simulink model "guidance_2016"  (R2016b)
settings: Solver=VariableStepAuto  StartTime=0.0  StopTime=1000.0  RelTol=1e-3
libraries: marine_gnc x1
settings Model: Creator=mikkelsorensen  LastModifiedBy=mikkelsorensen

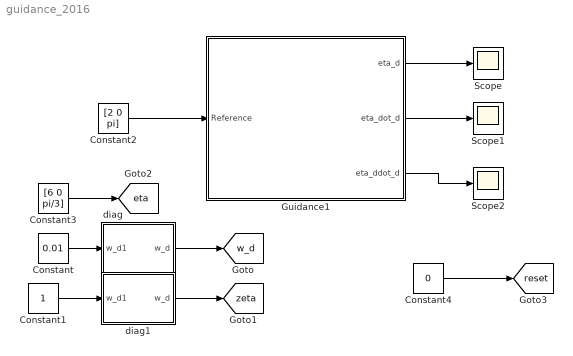
== system guidance_2016 ==
  Constant : Constant  Value=0.01
  Constant1 : Constant
  Constant2 : Constant  Value=[2 0 pi]
  Constant3 : Constant  Value=[6 0 pi/3]
  Constant4 : Constant  Value=0
  Guidance1 : Subsystem
  Scope : Scope
  Scope1 : Scope
  Scope2 : Scope
  diag : MATLAB Function  TreatAsAtomicUnit=on
  diag1 : MATLAB Function  TreatAsAtomicUnit=on
  tag scope: eta=global, reset=global, w_d=global, zeta=global
  wires:
  Constant/1 -> diag/1(w_d1)
  Constant1/1 -> diag1/1(w_d1)
  Constant2/1 -> Guidance1/1("Reference ")
  Constant3/1 -> [eta]
  Constant4/1 -> [reset]
  diag/1(w_d) -> [w_d]
  diag1/1(w_d) -> [zeta]
  Guidance1/1(eta_d) -> Scope/1
  Guidance1/3(eta_ddot_d) -> Scope2/1
  Guidance1/2(eta_dot_d) -> Scope1/1

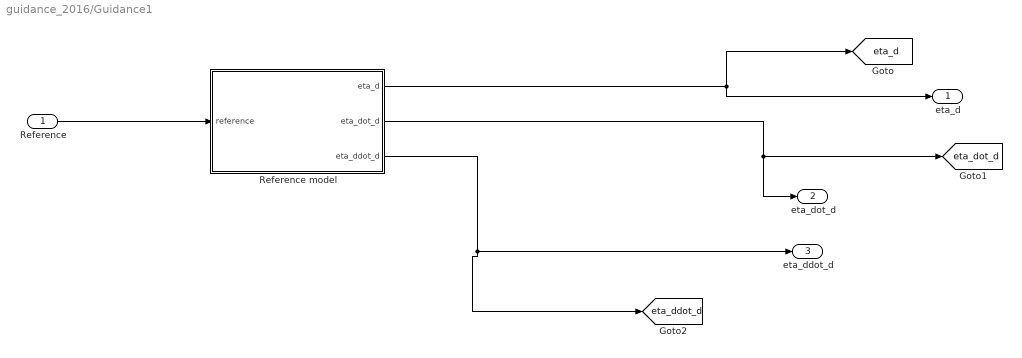
== system guidance_2016/Guidance1 ==
  "Reference " : Inport
  Reference model : Subsystem
  eta_d : Outport
  eta_dot_d : Outport  Port=2
  eta_ddot_d : Outport  Port=3
  tag scope: eta_d=global, eta_ddot_d=global, eta_dot_d=global
  wires:
  Reference model/1(eta_d) -> [eta_d], eta_d/1
  Reference model/2(eta_dot_d) -> eta_dot_d/1, [eta_dot_d]
  Reference model/3(eta_ddot_d) -> [eta_ddot_d], eta_ddot_d/1
  "Reference "/1 -> Reference model/1(reference)

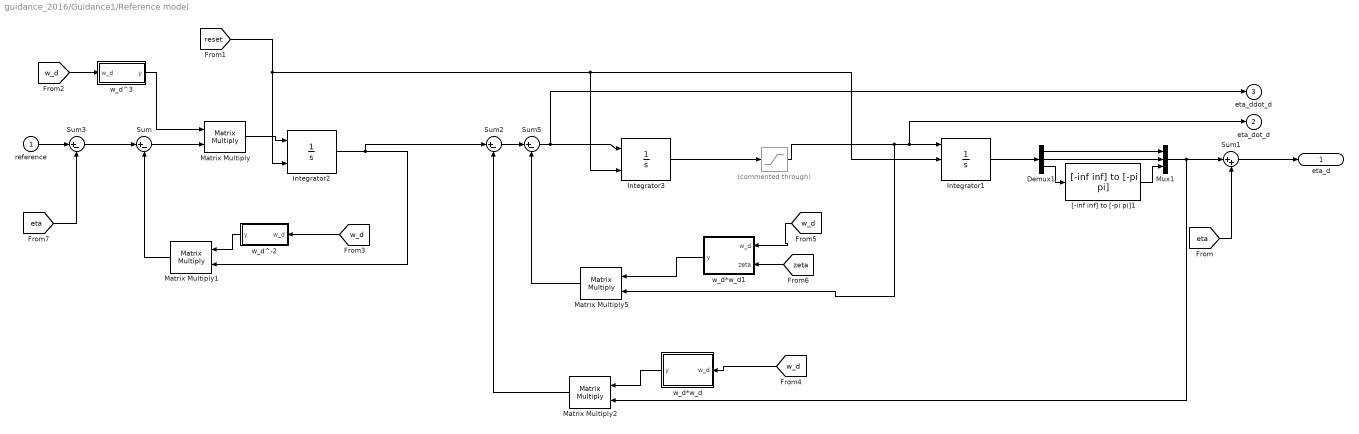
== system guidance_2016/Guidance1/Reference model ==
  reference : Inport
  "       " : Saturate  Commented=through  UpperLimit=[0.3 0.1 1]  LowerLimit=-[0.3 0.1 1]
  Demux1 : Demux  Outputs=3
  Integrator1 : Integrator  ExternalReset=either  InitialConditionSource=external
  Integrator2 : Integrator  ExternalReset=either
  Integrator3 : Integrator  ExternalReset=either
  Matrix Multiply{,1..2,5} (4 alike) : Product  Multiplication=Matrix(*)
  Mux1 : Mux  Inputs=3
  Sum : Sum  Inputs=|+-
  Sum1 : Sum  Inputs=|++  SaturateOnIntegerOverflow=on  InputSameDT=on  OutDataTypeStr=Inherit: Same as first input
  Sum2 : Sum  Inputs=|+-  SaturateOnIntegerOverflow=on  InputSameDT=on  OutDataTypeStr=Inherit: Same as first input
  Sum3 : Sum  Inputs=|+-  SaturateOnIntegerOverflow=on  InputSameDT=on  OutDataTypeStr=Inherit: Same as first input
  Sum5 : Sum  Inputs=|+-  SaturateOnIntegerOverflow=on  InputSameDT=on  OutDataTypeStr=Inherit: Same as first input
  "[-inf inf] to [-pi pi]1" : marine_gnc/Utilities/Math Operations/[-inf inf] to [-pi pi]
  w_d*w_d : MATLAB Function  TreatAsAtomicUnit=on
  w_d*w_d1 : MATLAB Function  TreatAsAtomicUnit=on
  w_d^-2 : MATLAB Function  TreatAsAtomicUnit=on
  w_d^3 : MATLAB Function  TreatAsAtomicUnit=on
  eta_d : Outport  InitialOutput=0
  eta_dot_d : Outport  Port=2  InitialOutput=0
  eta_ddot_d : Outport  Port=3  InitialOutput=0
  wires:
  "       "/1 -> eta_dot_d/1, Integrator1/1, Matrix Multiply5/2
  Sum5/1 -> Integrator3/1, eta_ddot_d/1
  Integrator2/1 -> Sum2/1, Matrix Multiply1/2
  Sum2/1 -> Sum5/1
  Matrix Multiply2/1 -> Sum2/2
  Mux1/1 -> Sum1/1, Matrix Multiply2/2
  Integrator3/1 -> "       "/1
  Matrix Multiply5/1 -> Sum5/2
  Sum/1 -> Matrix Multiply/2
  Matrix Multiply/1 -> Integrator2/1
  Matrix Multiply1/1 -> Sum/2
  [w_d] -> w_d^3/1(w_d)
  [w_d] -> w_d^-2/1(w_d)
  [w_d] -> w_d*w_d/1(w_d)
  w_d*w_d/1(y) -> Matrix Multiply2/1
  [zeta] -> w_d*w_d1/2(zeta)
  [w_d] -> w_d*w_d1/1(w_d)
  w_d*w_d1/1(y) -> Matrix Multiply5/1
  [reset] -> Integrator3/2, Integrator1/2, Integrator2/2
  w_d^-2/1(y) -> Matrix Multiply1/1
  w_d^3/1(y) -> Matrix Multiply/1
  Demux1/1 -> Mux1/1
  "[-inf inf] to [-pi pi]1"/1 -> Mux1/3
  Demux1/3 -> "[-inf inf] to [-pi pi]1"/1
  Demux1/2 -> Mux1/2
  Integrator1/1 -> Demux1/1
  [eta] -> Sum1/2
  Sum1/1 -> eta_d/1
  reference/1 -> Sum3/1
  Sum3/1 -> Sum/1
  [eta] -> Sum3/2

== matlab function guidance_2016/diag1 ==
  data: w_d output; w_d1 input
function w_d = fcn(w_d1)
%#codegen

w_d = diag([w_d1,w_d1,w_d1]);

== matlab function guidance_2016/Guidance1/Reference model/w_d*w_d ==
  data: w_d input; y output
function y = fcn(w_d)
%#codegen

y = w_d*w_d;

== matlab function guidance_2016/diag ==
  data: w_d output; w_d1 input
function w_d = fcn(w_d1)
%#codegen

w_d = diag([w_d1,w_d1,w_d1]);

== matlab function guidance_2016/Guidance1/Reference model/w_d*w_d1 ==
  data: w_d input; y output; zeta input
function y = fcn(w_d,zeta)
%#codegen

y = 2*zeta*w_d;

== matlab function guidance_2016/Guidance1/Reference model/w_d^-2 ==
  data: w_d input; y output
function y = fcn(w_d)
%#codegen

y = w_d^-2;

== matlab function guidance_2016/Guidance1/Reference model/w_d^3 ==
  data: w_d input; y output
function y = fcn(w_d)
%#codegen

y = w_d^3;
